simulink model "Activo_ideal"  (R2021a)
settings: Solver=ode4  StartTime=0.0  StopTime=ttotal  FixedStep=dtsim  RelTol=1e-3
values from neighbouring files (symbols this model uses):
  Edificio = ss(ssA,[ssB1 ssB2],ssC,[ssD1 ssD2])    [CasoI.m]    (also in CasoII.m; CasoIII.m)
  Referencia = struct()    [CasoI.m]    (also in CasoII.m; CasoIII.m; CasoIII_graficos.m = load(['CasoIII_Resultados/Maule/Maule60'],'Referencia').Refe; CasoII_graficos.m = load(['CasoII_Resultados/Maule/Maule60'],'Referencia').Refer)
  sys_kalman = sys_kalman(4:9,:)    [CasoI.m]    (also in CasoII.m; CasoIII.m)
undefined symbols (not defined in the file or in its folder): Kc
settings Model: Creator=cristobal  LastModifiedBy=maryf
settings SolverCC: AlgebraicLoopSolver=TrustRegion
settings DataIOCC: ReturnWorkspaceOutputs=off
settings DebuggingCC: SFMachineParentedDataDiag=warning  ArithmeticOperatorsInVariantConditions=warning
settings SFSimCC: SimUseLocalCustomCode=off  CustomCodeUndefinedFunction=UseInterfaceOnly
settings RTWCC: RTWUseLocalCustomCode=off
settings CodeAppCC: StateflowObjectComments=on

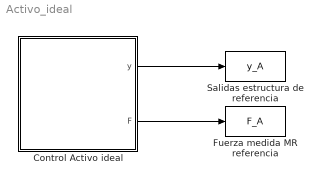
== system Activo_ideal ==
  Control Activo ideal : Subsystem
  Fuerza medida MR referencia : ToWorkspace  VariableName=F_A  SaveFormat=Timeseries  SampleTime=-1
  Salidas estructura de referencia : ToWorkspace  VariableName=y_A  SaveFormat=Timeseries  SampleTime=-1
  wires:
  Control Activo ideal/2(F) -> Fuerza medida MR referencia/1
  Control Activo ideal/1(y) -> Salidas estructura de referencia/1

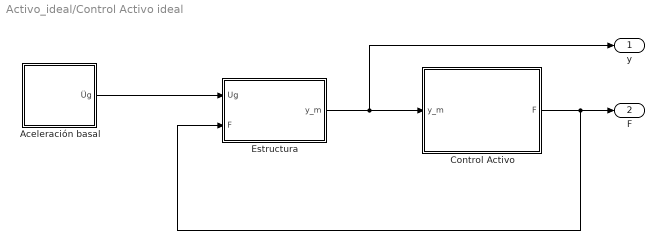
== system Activo_ideal/Control Activo ideal ==
  Aceleración basal : Subsystem
  Control Activo : Subsystem
  Estructura : Subsystem
  y : Outport  VectorParamsAs1DForOutWhenUnconnected=off
  F : Outport  Port=2  VectorParamsAs1DForOutWhenUnconnected=off
  wires:
  Control Activo/1(F) -> F/1, Estructura/2("F ")
  Estructura/1(y_m) -> y/1, Control Activo/1(y_m)
  Aceleración basal/1(Üg) -> Estructura/1(Ug)

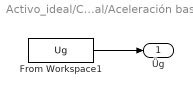
== system Activo_ideal/Control Activo ideal/Aceleración basal ==
  From Workspace1 : FromWorkspace  VariableName=Ug  OutputAfterFinalValue=Setting to zero
  Üg : Outport  VectorParamsAs1DForOutWhenUnconnected=off
  wires:
  From Workspace1/1 -> Üg/1

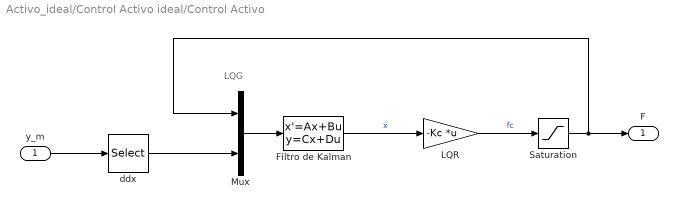
== system Activo_ideal/Control Activo ideal/Control Activo ==
  note: LQG
  y_m : Inport
  Filtro de Kalman : StateSpace  A=sys_kalman.a  B=sys_kalman.b  C=sys_kalman.c  D=sys_kalman.d  InitialCondition=0
  LQR : Gain  Gain=-Kc  Multiplication=Matrix(K*u) (u vector)
  Mux : Mux  Inputs=2
  Saturation : Saturate  UpperLimit=max(abs(Referencia.LQGCOC.F))  LowerLimit=-max(abs(Referencia.LQGCOC.F))
  ddx : Selector  InputPortWidth=12  IndexOptions=Index vector (dialog)  Indices=10:12  OutputSizes=1
  F : Outport
  wires:
  y_m/1 -> ddx/1
  LQR/1 -> Saturation/1  "fc"
  Mux/1 -> Filtro de Kalman/1
  ddx/1 -> Mux/2
  Filtro de Kalman/1 -> LQR/1  "x"
  Saturation/1 -> Mux/1, F/1

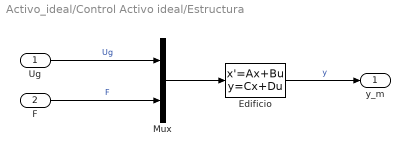
== system Activo_ideal/Control Activo ideal/Estructura ==
  Ug : Inport
  "F " : Inport  Port=2
  Edificio : StateSpace  A=Edificio.A  B=Edificio.B  C=Edificio.C  D=Edificio.D  InitialCondition=0
  Mux : Mux  Inputs=2
  y_m : Outport
  wires:
  Edificio/1 -> y_m/1  "y"
  Mux/1 -> Edificio/1
  Ug/1 -> Mux/1  "Ug"
  "F "/1 -> Mux/2  "F"
